simulink model "Simple_Model_Packaging_2"  (R2022b)
settings: Solver=VariableStepAuto  StartTime=0.0  StopTime=0.3  RelTol=1e-3
InitFcn:
  | Parameter_Initialize_2
undefined symbols (not defined in the file or in its folder): doppler, gcbh, magnitude, model, rcfiltgaincompat, rsgenpoly
libraries: commdigbbndpm3 x6, commfilt2 x6, simulink x5, commdigbbndam3 x4, commchan3 x3, commrandsrc3 x3, commblkcod2 x2, commblkintrlv2 x2, commofdm x2, commmimo x2, commseqgen3 x2, commsink2 x1
(part 1 of 2)
settings Model: Creator=89778  LastModifiedBy=79327

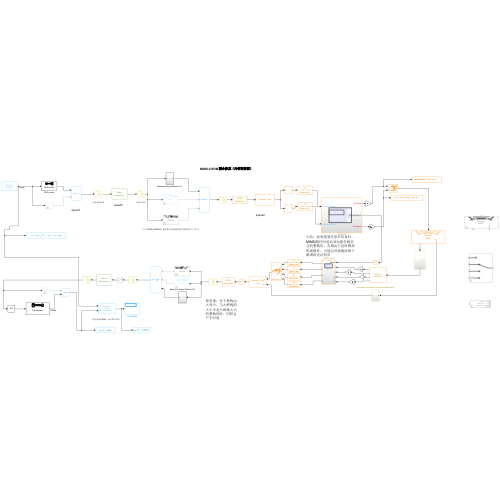
[thumbnail: Simulink's stored preview of the top-level diagram]
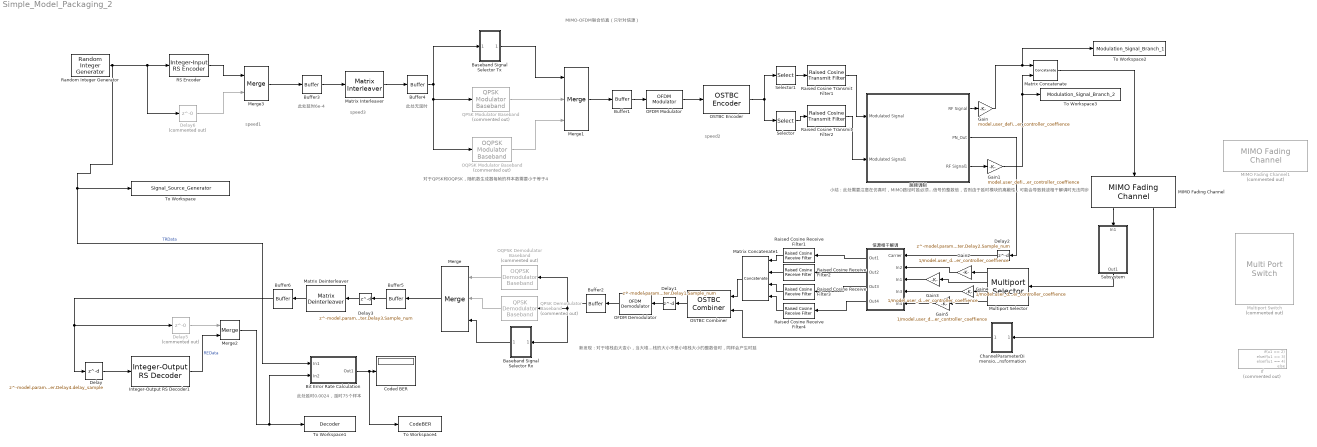
== system Simple_Model_Packaging_2 ==
  note: speed2
  note: 对于QPSK和OQPSK，随机数生成器每帧的样本数需要小于等于4
  note: MIMO-OFDM联合仿真（只针对信源）
  note: 此处延时6e-4
  note: 此处无延时
  note: 此处延时0.0024，延时75个样本
  note: 新发现：对于堆栈由大变小，当大堆栈的大小不是小堆栈大小的整数倍时，同样会产生时延
  note: 小结：此处需要注意在仿真时，MIMO路径时延必须为蓝色线信号的整数倍，否则由于延时模块的离散性，可能会导致载波相干解调时无法同步
  note: speed1
  note: speed3
  Baseband Signal Selector Rx : Subsystem
  Baseband Signal Selector Tx : Subsystem
  Bit Error Rate Calculation : Subsystem
      mask Display:
      | disp('Bit Error\nRate\nCalculation')
      | port_label('input', 1, 'Tx')
      | port_label('input', 2, 'Rx')
  Buffer1 : Buffer  N=model.parameter.Buffer1.Output_size  OutputFrames=off
  Buffer2 : Buffer  N=model.parameter.Buffer2.Output_buffer_size  OutputFrames=off
  Buffer3 : Buffer  N=model.parameter.Buffer3.Output_size  OutputFrames=off
  Buffer4 : Buffer  N=model.parameter.Buffer4.Output_size  OutputFrames=off
  Buffer5 : Buffer  N=model.parameter.Buffer5.Output_buffer_size  OutputFrames=off
  Buffer6 : Buffer  N=model.parameter.Buffer6.Output_buffer_size  OutputFrames=off
  ChannelParameterDimensionTransformation : Subsystem
  Coded BER : Display
  Delay : Delay  DelayLength=model.parameter.Delay4.delay_sample  InitialCondition=0  InputProcessing=Columns as channels (frame based)
  Delay1 : Delay  DelayLength=model.parameter.Delay1.Sample_num  InitialCondition=0  InputProcessing=Columns as channels (frame based)
  Delay2 : Delay  DelayLength=model.parameter.Delay2.Sample_num  InitialCondition=0  InputProcessing=Columns as channels (frame based)
  Delay3 : Delay  DelayLength=model.parameter.Delay3.Sample_num  InitialCondition=0  InputProcessing=Columns as channels (frame based)
  Delay5 : Delay  Commented=on  DelayLength=0  InitialCondition=0  InputProcessing=Columns as channels (frame based)
  Delay6 : Delay  Commented=on  DelayLength=0  InitialCondition=0
  Gain : Gain  Gain=model.user_defined.TR.Sig_power_controller_coeffience
  Gain1 : Gain  Gain=model.user_defined.TR.Sig_power_controller_coeffience
  Gain{2..5} (4 alike) : Gain  Gain=1/model.user_defined.TR.Sig_power_controller_coeffience
  If : If  Commented=on  IfExpression=u1 == 2  ElseIfExpressions=u1 == 3, u1 == 4
  Integer-Output RS Decoder1 : commblkcod2/Integer-Output RS Decoder  n=model.parameter.Integer_Output_RS_Decoder1.Codeword_Length  k=model.parameter.Integer_Output_RS_Decoder1.Message_Length  specShortening=off  shortenedK=3  specGenPoly=off  genPoly=rsgenpoly(7, 3, [], [], 'double')  specPrimPoly=off  prPoly='X^3 + X + 1'  specPuncture=off  punctVec=[ones(2,1); zeros(2,1)]  specErasurePort=off  showNumErr=off
  MIMO Fading Channel : commchan3/MIMO Fading Channel  InheritSampleRate=on  SampleRate=1  PathDelays=model.parameter.MIMO_Fading_Channel.Discrete_path_delays  AveragePathGains=model.parameter.MIMO_Fading_Channel.Average_path_gains  NormalizePathGains=on  FadingDistribution=Rayleigh  KFactor=3  DirectPathDopplerShift=0  DirectPathInitialPhase=0  MaximumDopplerShift=model.parameter.MIMO_Fading_Channel.Maximum_Doppler_shift  DopplerSpectrum=doppler('Jakes')  SpatialCorrelationSpecification=None  SpatialCorrelationMatrix=[1 0 0 0; 0 1 0 0; 0 0 1 0; 0 0 0 1]  NumTransmitAntennas=model.parameter.MIMO_Fading_Channel.TA_num  NumReceiveAntennas=model.parameter.MIMO_Fading_Channel.RA_num  TransmitCorrelationMatrix=[1 0; 0 1]  ReceiveCorrelationMatrix=[1 0; 0 1]  AntennaSelection=Off  NormalizeChannelOutputs=on  PathGainsOutputPort=on  SimulateUsing=Interpreted execution  FadingTechnique=Filtered Gaussian noise  NumSinusoids=48  InitialTimeSource=Property  InitialTime=0  RandomStream=mt19937ar with seed  Seed=73  Visualization=Off  AntennaPairsToDisplay=[ 1, 1 ]  PathsForDopplerDisplay=1  SamplesToDisplay=25%
  MIMO Fading Channel1 : commchan3/MIMO Fading Channel  Commented=on  InheritSampleRate=on  SampleRate=1  PathDelays=[0.000265 0.000265*5]  AveragePathGains=[5 5]  NormalizePathGains=on  FadingDistribution=Rayleigh  KFactor=3  DirectPathDopplerShift=0  DirectPathInitialPhase=0  MaximumDopplerShift=50  DopplerSpectrum=doppler('Jakes')  SpatialCorrelationSpecification=None  SpatialCorrelationMatrix=[1 0 0 0; 0 1 0 0; 0 0 1 0; 0 0 0 1]  NumTransmitAntennas=2  NumReceiveAntennas=2  TransmitCorrelationMatrix=[1 0; 0 1]  ReceiveCorrelationMatrix=[1 0; 0 1]  AntennaSelection=Off  NormalizeChannelOutputs=on  PathGainsOutputPort=on  SimulateUsing=Interpreted execution  FadingTechnique=Filtered Gaussian noise  NumSinusoids=48  InitialTimeSource=Property  InitialTime=0  RandomStream=mt19937ar with seed  Seed=73  Visualization=Off  AntennaPairsToDisplay=[ 1, 1 ]  PathsForDopplerDisplay=1  SamplesToDisplay=25%
  Matrix Concatenate : Concatenate  NumInputs=model.parameter.Matrix_Concatenate.Input_num  Mode=Multidimensional array  ConcatenateDimension=model.parameter.Matrix_Concatenate.Cascade_Dimension
  Matrix Concatenate1 : Concatenate  NumInputs=model.parameter.Matrix_Concatenate1.Input_num  Mode=Multidimensional array  ConcatenateDimension=model.parameter.Matrix_Concatenate1.Cascade_Dimension
  Matrix Deinterleaver : commblkintrlv2/Matrix Deinterleaver  StatePerturbationForJacobian=1.0e-05  Nrows=model.parameter.Matrix_Deinterleaver.row_num  Ncols=model.parameter.Matrix_Deinterleaver.col_num
  Matrix Interleaver : commblkintrlv2/Matrix Interleaver  StatePerturbationForJacobian=1.0e-05  Nrows=model.parameter.Matrix_Interleaver.row_nums  Ncols=model.parameter.Matrix_Interleaver.col_nums
  Merge : Merge  Inputs=3
  Merge1 : Merge  Inputs=3
  Merge2 : Merge
  Merge3 : Merge
  Multiport Selector : dspindex/Multiport Selector  rowsOrCols=Columns  idxCellArray=model.parameter.Multiport_Selector.Indices_to_output  idxErrMode=Clip Index
  Multiport Switch : MultiPortSwitch  Commented=on  SaturateOnIntegerOverflow=off  InputSameDT=off
  OFDM Demodulator : commofdm/OFDM Demodulator  FFTLength=model.parameter.OFDM_Demodulator.FFT_length  NumGuardBandCarriers=model.parameter.OFDM_Demodulator.Number_of_guard_bands  RemoveDCCarrier=off  PilotOutputPort=off  PilotCarrierIndices=[12; 26; 40; 54]  CyclicPrefixLength=model.parameter.OFDM_Demodulator.Cyclic_prefix_length  NumSymbols=model.parameter.OFDM_Demodulator.Number_of_OFDM_symbols  NumReceiveAntennas=model.parameter.OFDM_Demodulator.Number_of_receive_antennas  SimulateUsing=Interpreted execution
  OFDM Modulator : commofdm/OFDM Modulator  StatePerturbationForJacobian=1.0e-05  FFTLength=model.parameter.OFDM_Modulator.FFT_length  NumGuardBandCarriers=model.parameter.OFDM_Modulator.guard_bands_num  InsertDCNull=off  PilotInputPort=off  PilotCarrierIndices=[12; 26; 40; 54]  CyclicPrefixLength=model.parameter.OFDM_Modulator.Cyclic_prefix_length  Windowing=off  WindowLength=1  NumSymbols=model.parameter.OFDM_Modulator.OFDM_symbols_num  NumTransmitAntennas=model.parameter.OFDM_Modulator.transmit_antennas_num  SimulateUsing=Interpreted execution
  OQPSK Demodulator Baseband : commdigbbndpm3/OQPSK Demodulator Baseband  Commented=on  OutType=Integer  Ph=0  Mapping=Gray  pulseShape=Half sine  num=[0.7071, 0.7071]  rolloff=0.2  filterSpan=10  sps=2  RateOptions=Enforce single-rate processing  outDtype2=double
  OQPSK Modulator Baseband : commdigbbndpm3/OQPSK Modulator Baseband  Commented=on  InType=Integer  Ph=0  Mapping=Gray  pulseShape=Half sine  num=[0.7071, 0.7071]  rolloff=0.2  filterSpan=10  sps=2  RateOptions=Enforce single-rate processing  outDtype=double
  OSTBC Combiner : commmimo/OSTBC Combiner  numTx=2  rate=3/4  numRx=4  roundingMode=Floor  overflowMode=Wrap  OvFlMode=off  OvFlModeLastStrValue=off  crossProductWordLen=32  crossProductFracLen=16  crossSumWordLen=32  crossSumFracLen=16  egyProductWordLen=32  egyProductFracLen=16  egySumWordLen=32  egySumFracLen=16  divisionWordLen=32  divisionFracLen=16  divisionDataTypeStr=Inherit: Same as accumulator  divisionLastDataTypeStr=Inherit: Same as accumulator
  OSTBC Encoder : commmimo/OSTBC Encoder  numTx=2  rate=3/4  overflowMode=Wrap  OvFlMode=off  OvFlModeLastStrValue=off
  QPSK Demodulator Baseband : commdigbbndpm3/QPSK Demodulator Baseband  Commented=on  OutType=Integer  DecType=Hard decision  VarSource=Dialog  Variance=1  Dec=Gray  Ph=pi/4  outDtype1=Inherit via internal rule  outDtype2=Inherit via internal rule  derotateFactorWordLen=16  derotateFactorDataTypeStr=Inherit: Same word length as input  derotateFactorLastDataTypeStr=Inherit: Same word length as input
  QPSK Modulator Baseband : commdigbbndpm3/QPSK Modulator Baseband  Commented=on  InType=Integer  Enc=Gray  Ph=pi/4  outDtype=double  outWordLen=16  outUDDataType=sfix(16)  outFracLenMode=Best precision  outFracLen=15  outDataTypeStr=double  outLastDataTypeStr=double
  RS Encoder : commblkcod2/Integer-Input RS Encoder  n=model.parameter.RS_Encoder.Codeword_Length  k=model.parameter.RS_Encoder.Message_Length  specShortening=off  shortenedK=3  specGenPoly=off  genPoly=rsgenpoly(7,3)  specPrimPoly=off  prPoly=[1 0 1 1]  specPuncture=off  punctVec=[ones(2,1); zeros(2,1)]
  Raised Cosine Receive Filter1 : commfilt2/Raised Cosine Receive Filter  filtType=Square root  R=model.parameter.Raised_Cosine_Receive_Filter1.Rolloff_factor  filtSpan=model.parameter.Raised_Cosine_Receive_Filter1.Filter_span_in_symbols  N=model.parameter.Raised_Cosine_Receive_Filter1.Input_samples_per_symbol  downFactor=model.parameter.Raised_Cosine_Receive_Filter1.Decimation_factor  downOffset=0  filterGain=rcfiltgaincompat(gcbh)  InputProcessing=Columns as channels (frame based)  RateOptions=Enforce single-rate processing  framing=Mute  checkCoeff=off  variableName=rcRxFilt1  currentFiltSpan=10  D=5  inputOffset=0  sampMode=Mute  saveAsFlag=0  rateMode=Downsampling  checkGain=Normalized  launchFVT=on  roundingMode=Floor  overflowMode=off  coeffDataTypeStr=Inherit: Same word length as input  coeffMin=[]  coeffMax=[]  coeffLastDataTypeStr=Inherit: Same word length as input  accumDataTypeStr=Inherit: Same as product output  accumLastDataTypeStr=Inherit: Same as product output  outputDataTypeStr=Inherit: Same as accumulator  outputMin=[]  outputMax=[]  outputLastDataTypeStr=Inherit: Same as accumulator
  Raised Cosine Receive Filter2 : commfilt2/Raised Cosine Receive Filter  filtType=Square root  R=model.parameter.Raised_Cosine_Receive_Filter2.Rolloff_factor  filtSpan=model.parameter.Raised_Cosine_Receive_Filter2.Filter_span_in_symbols  N=model.parameter.Raised_Cosine_Receive_Filter2.Input_samples_per_symbol  downFactor=model.parameter.Raised_Cosine_Receive_Filter2.Decimation_factor  downOffset=0  filterGain=rcfiltgaincompat(gcbh)  InputProcessing=Columns as channels (frame based)  RateOptions=Enforce single-rate processing  framing=Mute  checkCoeff=off  variableName=rcRxFilt2  currentFiltSpan=10  D=5  inputOffset=0  sampMode=Mute  saveAsFlag=0  rateMode=Downsampling  checkGain=Normalized  launchFVT=on  roundingMode=Floor  overflowMode=off  coeffDataTypeStr=Inherit: Same word length as input  coeffMin=[]  coeffMax=[]  coeffLastDataTypeStr=Inherit: Same word length as input  accumDataTypeStr=Inherit: Same as product output  accumLastDataTypeStr=Inherit: Same as product output  outputDataTypeStr=Inherit: Same as accumulator  outputMin=[]  outputMax=[]  outputLastDataTypeStr=Inherit: Same as accumulator
  Raised Cosine Receive Filter3 : commfilt2/Raised Cosine Receive Filter  filtType=Square root  R=model.parameter.Raised_Cosine_Receive_Filter2.Rolloff_factor  filtSpan=model.parameter.Raised_Cosine_Receive_Filter2.Filter_span_in_symbols  N=model.parameter.Raised_Cosine_Receive_Filter2.Input_samples_per_symbol  downFactor=model.parameter.Raised_Cosine_Receive_Filter2.Decimation_factor  downOffset=0  filterGain=rcfiltgaincompat(gcbh)  InputProcessing=Columns as channels (frame based)  RateOptions=Enforce single-rate processing  framing=Mute  checkCoeff=off  variableName=rcRxFilt3  currentFiltSpan=10  D=5  inputOffset=0  sampMode=Mute  saveAsFlag=0  rateMode=Downsampling  checkGain=Normalized  launchFVT=on  roundingMode=Floor  overflowMode=off  coeffDataTypeStr=Inherit: Same word length as input  coeffMin=[]  coeffMax=[]  coeffLastDataTypeStr=Inherit: Same word length as input  accumDataTypeStr=Inherit: Same as product output  accumLastDataTypeStr=Inherit: Same as product output  outputDataTypeStr=Inherit: Same as accumulator  outputMin=[]  outputMax=[]  outputLastDataTypeStr=Inherit: Same as accumulator
  Raised Cosine Receive Filter4 : commfilt2/Raised Cosine Receive Filter  filtType=Square root  R=model.parameter.Raised_Cosine_Receive_Filter2.Rolloff_factor  filtSpan=model.parameter.Raised_Cosine_Receive_Filter2.Filter_span_in_symbols  N=model.parameter.Raised_Cosine_Receive_Filter2.Input_samples_per_symbol  downFactor=model.parameter.Raised_Cosine_Receive_Filter2.Decimation_factor  downOffset=0  filterGain=rcfiltgaincompat(gcbh)  InputProcessing=Columns as channels (frame based)  RateOptions=Enforce single-rate processing  framing=Mute  checkCoeff=off  variableName=rcRxFilt4  currentFiltSpan=10  D=5  inputOffset=0  sampMode=Mute  saveAsFlag=0  rateMode=Downsampling  checkGain=Normalized  launchFVT=on  roundingMode=Floor  overflowMode=off  coeffDataTypeStr=Inherit: Same word length as input  coeffMin=[]  coeffMax=[]  coeffLastDataTypeStr=Inherit: Same word length as input  accumDataTypeStr=Inherit: Same as product output  accumLastDataTypeStr=Inherit: Same as product output  outputDataTypeStr=Inherit: Same as accumulator  outputMin=[]  outputMax=[]  outputLastDataTypeStr=Inherit: Same as accumulator
  Raised Cosine Transmit Filter1 : commfilt2/Raised Cosine Transmit Filter  filtType=Square root  R=model.parameter.Raised_Cosine_Transmit_Filter1.Rolloff_factor  filtSpan=model.parameter.Raised_Cosine_Transmit_Filter1.Filter_span_in_symbols  N=model.parameter.Raised_Cosine_Transmit_Filter1.Output_samples_per_symbol  filterGain=rcfiltgaincompat(gcbh)  InputProcessing=Columns as channels (frame based)  RateOptions=Enforce single-rate processing  framing=Mute  checkCoeff=off  variableName=rcTxFilt1  checkGain=Normalized  sampMode=Mute  saveAsFlag=0  currentFiltSpan=10  D=(10)/2  launchFVT=on  roundingMode=Floor  overflowMode=off  coeffDataTypeStr=Inherit: Same word length as input  coeffMin=[]  coeffMax=[]  coeffLastDataTypeStr=Inherit: Same word length as input  outputDataTypeStr=Inherit: Same as accumulator  outputMin=[]  outputMax=[]  outputLastDataTypeStr=Inherit: Same as accumulator
  Raised Cosine Transmit Filter2 : commfilt2/Raised Cosine Transmit Filter  filtType=Square root  R=model.parameter.Raised_Cosine_Transmit_Filter2.Rolloff_factor  filtSpan=model.parameter.Raised_Cosine_Transmit_Filter2.Filter_span_in_symbols  N=model.parameter.Raised_Cosine_Transmit_Filter2.Output_samples_per_symbol  filterGain=rcfiltgaincompat(gcbh)  InputProcessing=Columns as channels (frame based)  RateOptions=Enforce single-rate processing  framing=Mute  checkCoeff=off  variableName=rcTxFilt2  checkGain=Normalized  sampMode=Mute  saveAsFlag=0  currentFiltSpan=10  D=(10)/2  launchFVT=on  roundingMode=Floor  overflowMode=off  coeffDataTypeStr=Inherit: Same word length as input  coeffMin=[]  coeffMax=[]  coeffLastDataTypeStr=Inherit: Same word length as input  outputDataTypeStr=Inherit: Same as accumulator  outputMin=[]  outputMax=[]  outputLastDataTypeStr=Inherit: Same as accumulator
  Random Integer Generator : commrandsrc3/Random Integer Generator  SetSize=model.parameter.Random_Integer_Generator.SetSize  SeedSource=Auto  Seed=4  SampleTime=model.parameter.Random_Integer_Generator.Random_Sample_Time  SamplesPerFrame=model.parameter.Random_Integer_Generator.Samples_per_frame  OutputDataType=double  SimulateUsing=Interpreted execution
  Selector : Selector  NumberOfDimensions=2  InputPortWidth=3  IndexOptions=Index vector (dialog),Index vector (dialog)  Indices=[1:272],2  OutputSizes=1,1
  Selector1 : Selector  NumberOfDimensions=2  InputPortWidth=3  IndexOptions=Index vector (dialog),Index vector (dialog)  Indices=[1:272],1  OutputSizes=1,1
  Subsystem : Subsystem
  To Workspace : ToWorkspace  VariableName=Signal_Source_Generator  SaveFormat=Timeseries  SampleTime=-1
  To Workspace1 : ToWorkspace  VariableName=Decoder  SaveFormat=Timeseries  SampleTime=-1
  To Workspace2 : ToWorkspace  VariableName=Modulation_Signal_Branch_1  SaveFormat=Timeseries  SampleTime=-1
  To Workspace3 : ToWorkspace  VariableName=Modulation_Signal_Branch_2  SaveFormat=Timeseries  SampleTime=-1
  To Workspace4 : ToWorkspace  VariableName=CodeBER  SaveFormat=Timeseries  SampleTime=-1
  信源相干解调 : Subsystem
  跳频调制 : Subsystem
  wires:
  Selector/1 -> Raised Cosine Transmit Filter2/1
  Selector1/1 -> Raised Cosine Transmit Filter1/1
  Matrix Interleaver/1 -> Buffer4/1
  Buffer3/1 -> Matrix Interleaver/1
  Buffer1/1 -> OFDM Modulator/1
  OFDM Modulator/1 -> OSTBC Encoder/1
  OSTBC Encoder/1 -> Selector1/1, Selector/1
  Raised Cosine Transmit Filter1/1 -> 跳频调制/1(Modulated Signal)
  Raised Cosine Transmit Filter2/1 -> 跳频调制/2(Modulated Signal1)
  跳频调制/1(RF Signal) -> Gain/1
  跳频调制/3(RF Signal1) -> Gain1/1
  Delay2/1 -> 信源相干解调/1(Carrier)
  信源相干解调/2(Out2) -> Raised Cosine Receive Filter2/1
  MIMO Fading Channel/2 -> ChannelParameterDimensionTransformation/1(In1)
  OFDM Demodulator/1 -> Buffer2/1
  Bit Error Rate Calculation/1(Out1) -> To Workspace4/1, Coded BER/1
  Raised Cosine Receive Filter1/1 -> Matrix Concatenate1/1
  Multiport Selector/1 -> Gain2/1
  Multiport Selector/2 -> Gain3/1
  Matrix Deinterleaver/1 -> Buffer6/1
  信源相干解调/1(Out1) -> Raised Cosine Receive Filter1/1
  OSTBC Combiner/1 -> Delay1/1
  Delay3/1 -> Matrix Deinterleaver/1
  Matrix Concatenate1/1 -> OSTBC Combiner/1
  ChannelParameterDimensionTransformation/1(Out1) -> OSTBC Combiner/2
  Raised Cosine Receive Filter2/1 -> Matrix Concatenate1/2
  Delay1/1 -> OFDM Demodulator/1
  跳频调制/2(PN_Out) -> Delay2/1
  MIMO Fading Channel/1 -> Subsystem/1(In1)
  Subsystem/1(Out1) -> Multiport Selector/1
  Multiport Selector/3 -> Gain4/1
  Multiport Selector/4 -> Gain5/1
  信源相干解调/3(Out3) -> Raised Cosine Receive Filter3/1
  信源相干解调/4(Out4) -> Raised Cosine Receive Filter4/1
  Raised Cosine Receive Filter3/1 -> Matrix Concatenate1/3
  Raised Cosine Receive Filter4/1 -> Matrix Concatenate1/4
  QPSK Modulator Baseband/1 -> Merge1/2
  Random Integer Generator/1 -> RS Encoder/1, Delay6/1, To Workspace/1, Bit Error Rate Calculation/1(In1)  "TRData"
  Baseband Signal Selector Tx/1(Out1) -> Merge1/1
  OQPSK Modulator Baseband/1 -> Merge1/3
  Delay5/1 -> Merge2/1
  Delay/1 -> Integer-Output RS Decoder1/1
  Integer-Output RS Decoder1/1 -> Merge2/2  "REData"
  Merge2/1 -> To Workspace1/1, Bit Error Rate Calculation/2(In2)
  Buffer4/1 -> Baseband Signal Selector Tx/1(In1), QPSK Modulator Baseband/1, OQPSK Modulator Baseband/1
  Merge1/1 -> Buffer1/1
  RS Encoder/1 -> Merge3/1
  Delay6/1 -> Merge3/2
  Merge3/1 -> Buffer3/1
  Buffer6/1 -> Delay/1, Delay5/1
  Buffer5/1 -> Delay3/1
  Buffer2/1 -> OQPSK Demodulator Baseband/1, Baseband Signal Selector Rx/1(In1), QPSK Demodulator Baseband/1
  OQPSK Demodulator Baseband/1 -> Merge/1
  QPSK Demodulator Baseband/1 -> Merge/2
  Baseband Signal Selector Rx/1(Out1) -> Merge/3
  Merge/1 -> Buffer5/1
  Gain/1 -> To Workspace2/1, Matrix Concatenate/1
  Gain1/1 -> Matrix Concatenate/2, To Workspace3/1
  Gain2/1 -> 信源相干解调/2(In2)
  Gain3/1 -> 信源相干解调/3(In1)
  Gain4/1 -> 信源相干解调/4(In3)
  Gain5/1 -> 信源相干解调/5(In4)
  Matrix Concatenate/1 -> MIMO Fading Channel/1

== system Simple_Model_Packaging_2/Baseband Signal Selector Rx ==
  In1 : Inport
  Constant : Constant  Value=model.user_defined.TR.Baseband_Modulation_type
  If : If  IfExpression=u1 == 1  ElseIfExpressions=u1 == 2
  If Action Subsystem1 : Subsystem  TreatAsAtomicUnit=on
  If Action Subsystem4 : Subsystem  TreatAsAtomicUnit=on
  If Action Subsystem5 : Subsystem  TreatAsAtomicUnit=on
  Merge : Merge  Inputs=3
  Out1 : Outport
  wires:
  In1/1 -> If Action Subsystem4/1(In1), If Action Subsystem1/1(In1), If Action Subsystem5/1(In1)
  If Action Subsystem5/1(Out1) -> Merge/3
  If Action Subsystem1/1(Out1) -> Merge/2
  If Action Subsystem4/1(Out1) -> Merge/1
  Constant/1 -> If/1
  Merge/1 -> Out1/1
  If/3 -> If Action Subsystem5/Action
  If/1 -> If Action Subsystem4/Action
  If/2 -> If Action Subsystem1/Action

== system Simple_Model_Packaging_2/Baseband Signal Selector Tx ==
  In1 : Inport
  Constant : Constant  Value=model.user_defined.TR.Baseband_Modulation_type
  If : If  IfExpression=u1 == 1  ElseIfExpressions=u1 == 2
  If Action Subsystem1 : Subsystem  TreatAsAtomicUnit=on
  If Action Subsystem4 : Subsystem  TreatAsAtomicUnit=on
  If Action Subsystem5 : Subsystem  TreatAsAtomicUnit=on
  Merge : Merge  Inputs=3
  Out1 : Outport
  wires:
  If Action Subsystem5/1(Out1) -> Merge/3
  Constant/1 -> If/1
  Merge/1 -> Out1/1
  If/3 -> If Action Subsystem5/Action
  If/1 -> If Action Subsystem4/Action
  If/2 -> If Action Subsystem1/Action
  If Action Subsystem1/1(Out1) -> Merge/2
  If Action Subsystem4/1(Out1) -> Merge/1
  In1/1 -> If Action Subsystem4/1(In1), If Action Subsystem1/1(In1), If Action Subsystem5/1(In1)

== system Simple_Model_Packaging_2/Bit Error Rate Calculation ==
  In1 : Inport
  In2 : Inport  Port=2
  Error Rate Calculation : commsink2/Error Rate Calculation  N=model.parameter.Error_Rate_Calculation.Receive_delay  st_delay=0  cp_mode=Entire frame  subframe=[]  PMode=Port  WsName=ErrorVec  RsMode2=off  stop=on  numErr=1e8  maxBits=1e10
  Integer to Bit Converter : simulink/Logic and Bit Operations/Integer to Bit Converter  nbits=model.parameter.Integer_to_Bit_Converter.M  signedInputValues=Unsigned  bitOrder=MSB first  outDtype=Inherit via internal rule
      settings: LibrarySourceBlock=|
      | commutil2/Integer to Bit
      | Converter
  Integer to Bit Converter1 : simulink/Logic and Bit Operations/Integer to Bit Converter  nbits=model.parameter.Integer_to_Bit_Converter1.M  signedInputValues=Unsigned  bitOrder=MSB first  outDtype=Inherit via internal rule
      settings: LibrarySourceBlock=|
      | commutil2/Integer to Bit
      | Converter
  Out1 : Outport  VectorParamsAs1DForOutWhenUnconnected=off
  wires:
  Integer to Bit Converter/1 -> Error Rate Calculation/1
  Integer to Bit Converter1/1 -> Error Rate Calculation/2
  In1/1 -> Integer to Bit Converter/1
  Error Rate Calculation/1 -> Out1/1
  In2/1 -> Integer to Bit Converter1/1

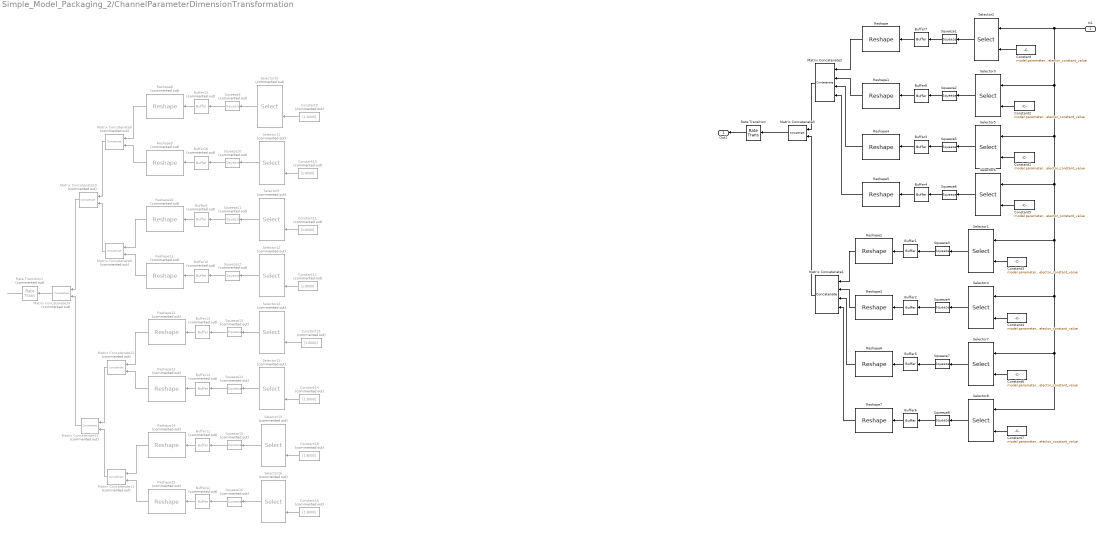
== system Simple_Model_Packaging_2/ChannelParameterDimensionTransformation ==
  In1 : Inport
  Buffer{1..8} (8 alike) : Buffer  N=model.parameter.CSI.buffers_length  OutputFrames=off
  Buffer{9..16} (8 alike) : Buffer  Commented=on  N=80  OutputFrames=off
  Constant{,1..7} (8 alike) : Constant  Value=model.parameter.CSI.selector_constant_value
  Constant{9..16} (8 alike) : Constant  Commented=on  Value=[1:8000]
  Matrix Concatenate1 : Concatenate  NumInputs=4  Mode=Multidimensional array  ConcatenateDimension=3
  Matrix Concatenate10 : Concatenate  Commented=on  Mode=Multidimensional array  ConcatenateDimension=3
  Matrix Concatenate{8..9,11..12} (4 alike) : Concatenate  Commented=on  Mode=Multidimensional array  ConcatenateDimension=4
  Matrix Concatenate13 : Concatenate  Commented=on  Mode=Multidimensional array  ConcatenateDimension=3
  Matrix Concatenate14 : Concatenate  Commented=on  Mode=Multidimensional array  ConcatenateDimension=2
  Matrix Concatenate2 : Concatenate  NumInputs=4  Mode=Multidimensional array  ConcatenateDimension=3
  Matrix Concatenate3 : Concatenate  Mode=Multidimensional array  ConcatenateDimension=2
  Rate Transition : RateTransition  OutPortSampleTime=model.Intermediate_variable.system_frame_speed_2
  Rate Transition1 : RateTransition  Commented=on  OutPortSampleTime=2.65e-4
  Reshape{,1..7} (8 alike) : Reshape  OutputDimensionality=Customize  OutputDimensions=model.parameter.CSI.reshape_dimension
  Reshape{8..15} (8 alike) : Reshape  Commented=on  OutputDimensionality=Customize  OutputDimensions=[80,1,1,1]
  Selector1 : Selector  NumberOfDimensions=4  InputPortWidth=3  IndexOptions=Index vector (port),Index vector (dialog),Index vector (dialog),Index vector (dialog)  Indices=[1 3],1,2,1  OutputSizes=1,1,1,1
  Selector10 : Selector  Commented=on  NumberOfDimensions=4  InputPortWidth=3  IndexOptions=Index vector (port),Index vector (dialog),Index vector (dialog),Index vector (dialog)  Indices=[1 3],1,1,1  OutputSizes=1,1,1,1
  Selector11 : Selector  Commented=on  NumberOfDimensions=4  InputPortWidth=3  IndexOptions=Index vector (port),Index vector (dialog),Index vector (dialog),Index vector (dialog)  Indices=[1 3],1,1,2  OutputSizes=1,1,1,1
  Selector12 : Selector  Commented=on  NumberOfDimensions=4  InputPortWidth=3  IndexOptions=Index vector (port),Index vector (dialog),Index vector (dialog),Index vector (dialog)  Indices=[1 3],1,2,2  OutputSizes=1,1,1,1
  Selector13 : Selector  Commented=on  NumberOfDimensions=4  InputPortWidth=3  IndexOptions=Index vector (port),Index vector (dialog),Index vector (dialog),Index vector (dialog)  Indices=[1 3],2,2,1  OutputSizes=1,1,1,1
  Selector14 : Selector  Commented=on  NumberOfDimensions=4  InputPortWidth=3  IndexOptions=Index vector (port),Index vector (dialog),Index vector (dialog),Index vector (dialog)  Indices=[1 3],2,1,1  OutputSizes=1,1,1,1
  Selector15 : Selector  Commented=on  NumberOfDimensions=4  InputPortWidth=3  IndexOptions=Index vector (port),Index vector (dialog),Index vector (dialog),Index vector (dialog)  Indices=[1 3],2,1,2  OutputSizes=1,1,1,1
  Selector16 : Selector  Commented=on  NumberOfDimensions=4  InputPortWidth=3  IndexOptions=Index vector (port),Index vector (dialog),Index vector (dialog),Index vector (dialog)  Indices=[1 3],2,2,2  OutputSizes=1,1,1,1
  Selector2 : Selector  NumberOfDimensions=4  InputPortWidth=3  IndexOptions=Index vector (port),Index vector (dialog),Index vector (dialog),Index vector (dialog)  Indices=[1 3],1,1,1  OutputSizes=1,1,1,1
  Selector3 : Selector  NumberOfDimensions=4  InputPortWidth=3  IndexOptions=Index vector (port),Index vector (dialog),Index vector (dialog),Index vector (dialog)  Indices=[1 3],1,1,2  OutputSizes=1,1,1,1
  Selector4 : Selector  NumberOfDimensions=4  InputPortWidth=3  IndexOptions=Index vector (port),Index vector (dialog),Index vector (dialog),Index vector (dialog)  Indices=[1 3],1,2,2  OutputSizes=1,1,1,1
  Selector5 : Selector  NumberOfDimensions=4  InputPortWidth=3  IndexOptions=Index vector (port),Index vector (dialog),Index vector (dialog),Index vector (dialog)  Indices=[1 3],1,1,3  OutputSizes=1,1,1,1
  Selector6 : Selector  NumberOfDimensions=4  InputPortWidth=3  IndexOptions=Index vector (port),Index vector (dialog),Index vector (dialog),Index vector (dialog)  Indices=[1 3],1,1,4  OutputSizes=1,1,1,1
  Selector7 : Selector  NumberOfDimensions=4  InputPortWidth=3  IndexOptions=Index vector (port),Index vector (dialog),Index vector (dialog),Index vector (dialog)  Indices=[1 3],1,2,3  OutputSizes=1,1,1,1
  Selector8 : Selector  NumberOfDimensions=4  InputPortWidth=3  IndexOptions=Index vector (port),Index vector (dialog),Index vector (dialog),Index vector (dialog)  Indices=[1 3],1,2,4  OutputSizes=1,1,1,1
  Selector9 : Selector  Commented=on  NumberOfDimensions=4  InputPortWidth=3  IndexOptions=Index vector (port),Index vector (dialog),Index vector (dialog),Index vector (dialog)  Indices=[1 3],1,2,1  OutputSizes=1,1,1,1
  Squeeze{1..8} (8 alike) : Squeeze
  Squeeze{9..16} (8 alike) : Squeeze  Commented=on
  Out1 : Outport
  wires:
  Buffer8/1 -> Reshape1/1
  Buffer7/1 -> Reshape/1
  Squeeze2/1 -> Buffer8/1
  Constant2/1 -> Selector3/2
  Selector3/1 -> Squeeze2/1
  Constant/1 -> Selector2/2
  Selector2/1 -> Squeeze1/1
  Reshape/1 -> Matrix Concatenate2/1
  Squeeze1/1 -> Buffer7/1
  Reshape1/1 -> Matrix Concatenate2/2
  Selector1/1 -> Squeeze3/1
  Constant3/1 -> Selector1/2
  Squeeze3/1 -> Buffer1/1
  Selector4/1 -> Squeeze4/1
  Constant4/1 -> Selector4/2
  Squeeze4/1 -> Buffer2/1
  Buffer1/1 -> Reshape2/1
  Buffer2/1 -> Reshape3/1
  Reshape2/1 -> Matrix Concatenate1/1
  Reshape3/1 -> Matrix Concatenate1/2
  Matrix Concatenate2/1 -> Matrix Concatenate3/1
  Matrix Concatenate1/1 -> Matrix Concatenate3/2
  Rate Transition/1 -> Out1/1
  Matrix Concatenate3/1 -> Rate Transition/1
  Matrix Concatenate8/1 -> Matrix Concatenate10/2
  Squeeze12/1 -> Buffer10/1
  Buffer10/1 -> Reshape11/1
  Constant12/1 -> Selector12/2
  Reshape9/1 -> Matrix Concatenate9/2
  Buffer16/1 -> Reshape9/1
  Selector9/1 -> Squeeze11/1
  Reshape10/1 -> Matrix Concatenate8/1
  Reshape8/1 -> Matrix Concatenate9/1
  Buffer9/1 -> Reshape10/1
  Matrix Concatenate10/1 -> Matrix Concatenate14/1
  Buffer15/1 -> Reshape8/1
  Selector10/1 -> Squeeze9/1
  Constant9/1 -> Selector10/2
  Constant11/1 -> Selector9/2
  Constant10/1 -> Selector11/2
  Constant14/1 -> Selector15/2
  Selector15/1 -> Squeeze14/1
  Squeeze9/1 -> Buffer15/1
  Selector16/1 -> Squeeze16/1
  Selector13/1 -> Squeeze15/1
  Reshape15/1 -> Matrix Concatenate11/2
  Squeeze13/1 -> Buffer13/1
  Selector11/1 -> Squeeze10/1
  Squeeze14/1 -> Buffer14/1
  Buffer14/1 -> Reshape13/1
  Selector14/1 -> Squeeze13/1
  Buffer13/1 -> Reshape12/1
  Buffer11/1 -> Reshape14/1
  Matrix Concatenate13/1 -> Matrix Concatenate14/2
  Buffer12/1 -> Reshape15/1
  Matrix Concatenate11/1 -> Matrix Concatenate13/2
  Constant15/1 -> Selector13/2
  Squeeze16/1 -> Buffer12/1
  Squeeze10/1 -> Buffer16/1
  Reshape13/1 -> Matrix Concatenate12/2
  Matrix Concatenate9/1 -> Matrix Concatenate10/1
  Constant16/1 -> Selector16/2
  Constant13/1 -> Selector14/2
  Selector12/1 -> Squeeze12/1
  Rate Transition1/1 -> ?
  Reshape12/1 -> Matrix Concatenate12/1
  Squeeze15/1 -> Buffer11/1
  ? -> Selector9/1, Selector12/1, Selector16/1, Selector13/1, Selector15/1, Selector14/1, Selector11/1, Selector10/1
  Squeeze11/1 -> Buffer9/1
  Reshape11/1 -> Matrix Concatenate8/2
  Matrix Concatenate14/1 -> Rate Transition1/1
  Matrix Concatenate12/1 -> Matrix Concatenate13/1
  Reshape14/1 -> Matrix Concatenate11/1
  Constant1/1 -> Selector5/2
  Constant5/1 -> Selector6/2
  Squeeze5/1 -> Buffer3/1
  Buffer3/1 -> Reshape4/1
  Squeeze6/1 -> Buffer4/1
  Buffer4/1 -> Reshape5/1
  Selector5/1 -> Squeeze5/1
  Selector6/1 -> Squeeze6/1
  Reshape4/1 -> Matrix Concatenate2/3
  Reshape5/1 -> Matrix Concatenate2/4
  Selector7/1 -> Squeeze7/1
  Buffer5/1 -> Reshape6/1
  Squeeze7/1 -> Buffer5/1
  Constant6/1 -> Selector7/2
  In1/1 -> Selector6/1, Selector1/1, Selector8/1, Selector7/1, Selector4/1, Selector5/1, Selector3/1, Selector2/1
  Selector8/1 -> Squeeze8/1
  Buffer6/1 -> Reshape7/1
  Squeeze8/1 -> Buffer6/1
  Constant7/1 -> Selector8/2
  Reshape6/1 -> Matrix Concatenate1/3
  Reshape7/1 -> Matrix Concatenate1/4

== system Simple_Model_Packaging_2/Subsystem ==
  In1 : Inport
  AWGN Channel : commchan3/AWGN Channel  InputProcessing=Columns as channels (frame based)  seed=67  noiseMode="Signal to noise ratio  (SNR)"  EbNodB=10  EsNodB=10  SNRdB=model.parameter.Awgn.SNR  bitsPerSym=1  Ps=model.parameter.Awgn.input_power  Tsym=1  variance=1
  Add : Sum
  Buffer : Buffer  N=model.parameter.M_FSK_Modulator_Baseband1.Samples_per_symbol  OutputFrames=off
  NosieGen : Subsystem
  Vector Concatenate : Concatenate  NumInputs=4  Mode=Multidimensional array  ConcatenateDimension=2
  Out1 : Outport
  wires:
  In1/1 -> Add/2
  AWGN Channel/1 -> Out1/1
  Add/1 -> AWGN Channel/1  "RESignal"
  Vector Concatenate/1 -> Add/1
  Buffer/1 -> Vector Concatenate/4, Vector Concatenate/3, Vector Concatenate/2, Vector Concatenate/1  "TRSignal"
  NosieGen/1(Jamming_Signal_Output) -> Buffer/1

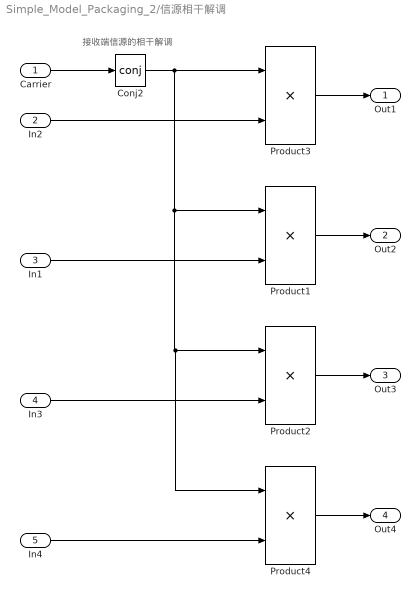
== system Simple_Model_Packaging_2/信源相干解调 ==
  note: 接收端信源的相干解调
  Carrier : Inport
  In2 : Inport  Port=2
  In1 : Inport  Port=3
  In3 : Inport  Port=4
  In4 : Inport  Port=5
  Conj2 : Math  Operator=conj
  Product{1..4} (4 alike) : Product
  Out1 : Outport
  Out2 : Outport  Port=2
  Out3 : Outport  Port=3
  Out4 : Outport  Port=4
  wires:
  Carrier/1 -> Conj2/1
  In2/1 -> Product3/2
  Product3/1 -> Out1/1
  In1/1 -> Product1/2
  Product1/1 -> Out2/1
  Conj2/1 -> Product4/1, Product2/1, Product1/1, Product3/1
  Product2/1 -> Out3/1
  Product4/1 -> Out4/1
  In3/1 -> Product2/2
  In4/1 -> Product4/2

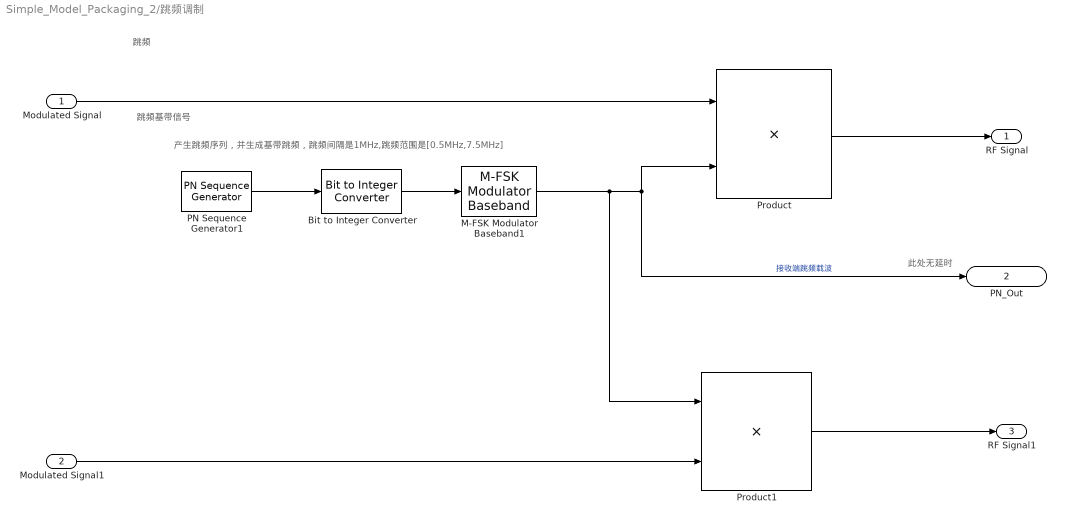
== system Simple_Model_Packaging_2/跳频调制 ==
  note: 跳频
  note: 此处无延时
  note: 跳频基带信号
  note: 产生跳频序列，并生成基带跳频，跳频间隔是1MHz,跳频范围是[0.5MHz,7.5MHz]
  Modulated Signal : Inport
  Modulated Signal1 : Inport  Port=2
  Bit to Integer Converter : simulink/Logic and Bit Operations/Bit to Integer Converter  nbits=model.parameter.Bit_to_Integer_Converter.M  bitOrder=MSB first  signedOutputValues=Unsigned  outDtype=double  outDtypeSigned=Inherit via internal rule
  M-FSK Modulator Baseband1 : commdigbbndfm2/M-FSK Modulator Baseband  M=model.parameter.M_FSK_Modulator_Baseband1.M_ary_number  InType=Integer  Enc=Gray  freqSep=model.parameter.M_FSK_Modulator_Baseband1.Frequency_separation  phaseType=Continuous  numSamp=model.parameter.M_FSK_Modulator_Baseband1.Samples_per_symbol  RateOptions=Enforce single-rate processing  outDataType=double
  PN Sequence Generator1 : commseqgen3/PN Sequence Generator  poly=model.parameter.PN_Sequence_Generator1.Generator_polynomial  ini_sta=model.parameter.PN_Sequence_Generator1.Initial_states  outBitMaskSource=Dialog parameter  shift=0  outVarSiz=off  maxOutSizeMode=Dialog parameter  maxOutSize=[10 1]  Ts=model.parameter.PN_Sequence_Generator1.Sample_time  sampPerFrame=model.parameter.PN_Sequence_Generator1.Samples_per_frame  reset=off  bitPackedOutputs=off  outDataType=double  numPackedBits=5  bitPackDataSigned=off  bitPackedOutDType=double
  Product : Product
  Product1 : Product
  RF Signal : Outport
  PN_Out : Outport  Port=2
  RF Signal1 : Outport  Port=3
  wires:
  M-FSK Modulator Baseband1/1 -> PN_Out/1, Product/2, Product1/1  "接收端跳频载波"
  Product/1 -> RF Signal/1
  Product1/1 -> RF Signal1/1
  Modulated Signal1/1 -> Product1/2
  Modulated Signal/1 -> Product/1
  PN Sequence Generator1/1 -> Bit to Integer Converter/1
  Bit to Integer Converter/1 -> M-FSK Modulator Baseband1/1

== system Simple_Model_Packaging_2/Baseband Signal Selector Rx/If Action Subsystem1 ==
  In1 : Inport
  Action Port : ActionPort  ActionPortLabel=elseif(u1 == 2)
  M-PSK Demodulator Baseband : commdigbbndpm3/M-PSK Demodulator Baseband  M=model.user_defined.Rectangular_QAM_Modulator_Baseband.M_Number  OutType=Integer  DecType=Hard decision  VarSource=Dialog  Variance=1  Dec=Gray  Mapping=[0:7]  Ph=0  outDtype1=Inherit via internal rule  outDtype2=Inherit via internal rule  derotateFactorWordLen=16  derotateFactorDataTypeStr=Inherit: Same word length as input  derotateFactorLastDataTypeStr=Inherit: Same word length as input
  Out1 : Outport
  wires:
  In1/1 -> M-PSK Demodulator Baseband/1
  M-PSK Demodulator Baseband/1 -> Out1/1  "REData"

== system Simple_Model_Packaging_2/Baseband Signal Selector Rx/If Action Subsystem4 ==
  In1 : Inport
  Action Port : ActionPort  ActionPortLabel=if(u1 == 1)
  Rectangular QAM Demodulator Baseband : commdigbbndam3/Rectangular QAM Demodulator Baseband  M=model.user_defined.Rectangular_QAM_Modulator_Baseband.M_Number  OutType=Integer  DecType=Hard decision  VarSource=Dialog  Variance=1  Dec=Gray  Mapping=[0:15]  PowType=Min. distance between symbols  MinDist=model.parameter.Rectangular_QAM_Demodulator_Baseband.Minimum_distance  AvgPow=1  PeakPow=1  Ph=0  outDtype1=Inherit via internal rule  outDtype2=Inherit via internal rule  derotateFactorWordLen=16  derotateFactorDataTypeStr=Inherit: Same word length as input  derotateFactorLastDataTypeStr=Inherit: Same word length as input  denormFactorWordLen=16  denormFactorDataTypeStr=Inherit: Same word length as input  denormFactorLastDataTypeStr=Inherit: Same word length as input  prodOutWordLen=32  prodOutOverflowMode=Wrap  prodOutRoundingMode=Floor  prodOutOvFlMode=off  prodOutOvFlModeLastStrValue=off  sumWordLen=32
  Out1 : Outport
  wires:
  In1/1 -> Rectangular QAM Demodulator Baseband/1
  Rectangular QAM Demodulator Baseband/1 -> Out1/1  "REData"

== system Simple_Model_Packaging_2/Baseband Signal Selector Rx/If Action Subsystem5 ==
  In1 : Inport
  Action Port : ActionPort  ActionPortLabel=else
  Rectangular QAM Demodulator Baseband : commdigbbndam3/Rectangular QAM Demodulator Baseband  M=model.user_defined.Rectangular_QAM_Modulator_Baseband.M_Number  OutType=Integer  DecType=Hard decision  VarSource=Dialog  Variance=1  Dec=Gray  Mapping=[0:15]  PowType=Min. distance between symbols  MinDist=2  AvgPow=1  PeakPow=1  Ph=0  outDtype1=Inherit via internal rule  outDtype2=Inherit via internal rule  derotateFactorWordLen=16  derotateFactorDataTypeStr=Inherit: Same word length as input  derotateFactorLastDataTypeStr=Inherit: Same word length as input  denormFactorWordLen=16  denormFactorDataTypeStr=Inherit: Same word length as input  denormFactorLastDataTypeStr=Inherit: Same word length as input  prodOutWordLen=32  prodOutOverflowMode=Wrap  prodOutRoundingMode=Floor  prodOutOvFlMode=off  prodOutOvFlModeLastStrValue=off  sumWordLen=32
  Out1 : Outport
  wires:
  In1/1 -> Rectangular QAM Demodulator Baseband/1
  Rectangular QAM Demodulator Baseband/1 -> Out1/1

== system Simple_Model_Packaging_2/Baseband Signal Selector Tx/If Action Subsystem1 ==
  In1 : Inport
  Action Port : ActionPort  ActionPortLabel=elseif(u1 == 2)
  M-PSK Modulator Baseband : commdigbbndpm3/M-PSK Modulator Baseband  M=model.user_defined.Rectangular_QAM_Modulator_Baseband.M_Number  InType=Integer  Enc=Gray  Mapping=[0:7]  Ph=0  outDtype=double  outWordLen=16  outUDDataType=sfix(16)  outFracLenMode=Best precision  outFracLen=15  outDataTypeStr=double  outLastDataTypeStr=double
  Out1 : Outport
  wires:
  M-PSK Modulator Baseband/1 -> Out1/1
  In1/1 -> M-PSK Modulator Baseband/1

== system Simple_Model_Packaging_2/Baseband Signal Selector Tx/If Action Subsystem4 ==
  In1 : Inport
  Action Port : ActionPort  ActionPortLabel=if(u1 == 1)
  Rectangular QAM Modulator Baseband : commdigbbndam3/Rectangular QAM Modulator Baseband  M=model.user_defined.Rectangular_QAM_Modulator_Baseband.M_Number  InType=Integer  Enc=Gray  Mapping=[0:15]  PowType=Min. distance between symbols  MinDist=model.parameter.Rectangular_QAM_Modulator_Baseband.Minimum_distance  AvgPow=1  PeakPow=1  Ph=0  outDtype=double  outWordLen=16  outUDDataType=sfix(16)  outFracLenMode=Best precision  outFracLen=15  outDataTypeStr=double  outLastDataTypeStr=double
      settings: LibrarySourceBlock=|
      | commhdldigbbndam/Rectangular QAM
      | Modulator
      | Baseband
  Out1 : Outport
  wires:
  Rectangular QAM Modulator Baseband/1 -> Out1/1
  In1/1 -> Rectangular QAM Modulator Baseband/1

== system Simple_Model_Packaging_2/Baseband Signal Selector Tx/If Action Subsystem5 ==
  In1 : Inport
  Action Port : ActionPort  ActionPortLabel=else
  Rectangular QAM Modulator Baseband1 : commdigbbndam3/Rectangular QAM Modulator Baseband  M=model.user_defined.Rectangular_QAM_Modulator_Baseband.M_Number  InType=Integer  Enc=Gray  Mapping=[0:15]  PowType=Min. distance between symbols  MinDist=2  AvgPow=1  PeakPow=1  Ph=0  outDtype=double  outWordLen=16  outUDDataType=sfix(16)  outFracLenMode=Best precision  outFracLen=15  outDataTypeStr=double  outLastDataTypeStr=double
      settings: LibrarySourceBlock=|
      | commhdldigbbndam/Rectangular QAM
      | Modulator
      | Baseband
  Out1 : Outport
  wires:
  In1/1 -> Rectangular QAM Modulator Baseband1/1
  Rectangular QAM Modulator Baseband1/1 -> Out1/1

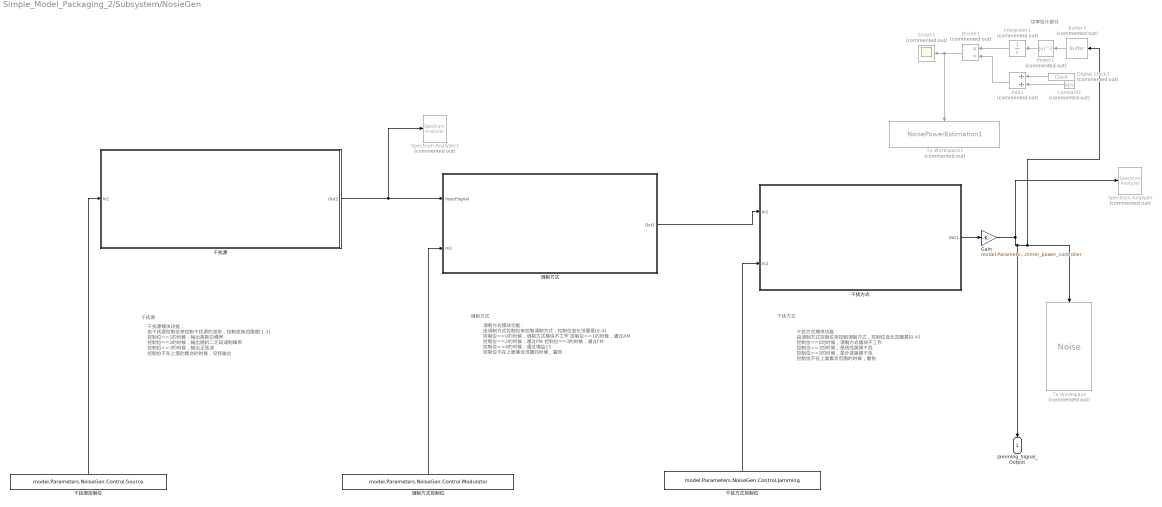
== system Simple_Model_Packaging_2/Subsystem/NosieGen ==
  note: 干扰源
  note: 调制方式
  note: 调制方式模块功能：
      | 由调制方式控制位来控制调制方式，控制位变化范围是[0-4]
      | 控制位==0的时候，调制方式模块不工作
      | 控制位==1的时候，通过AM
      | 控制位==2的时候，通过PM
      | 控制位==3的时候，通过FM
      | 控制位==4的时候，通过增益15
      | 控制位不在上面集合范围的时候，警告
  note: 干扰方式模块功能：
      | 由调制方式控制位来控制调制方式，控制位变化范围是[0-4]
      | 控制位==0的时候，调制方式模块不工作
      | 控制位==1的时候，是线性跳频干扰
      | 控制位==2的时候，是步进跳频干扰
      | 控制位不在上面集合范围的时候，警告
  note: 干扰源模块功能：
      | 由干扰源控制位来控制干扰源的波形，控制变换范围是[1-3]
      | 控制位==1的时候，输出高斯白噪声
      | 控制位==2的时候，输出随机二元码调制噪声
      | 控制位==3的时候，输出正弦波
      | 控制位不在上面的集合的时候，没有输出
  note: 干扰方式
  note: 功率估计部分
  Add1 : Sum  Commented=on
  Buffer7 : Buffer  Commented=on  N=1  OutputFrames=off
  Constant1 : Constant  Commented=on  Value=eps  SampleTime=model.Parameters.NoiseGen.NoiseTs
  Digital Clock1 : DigitalClock  Commented=on  SampleTime=model.Parameters.NoiseGen.NoiseTs
  Divide1 : Product  Commented=on  Inputs=*/
  Gain : Gain  Gain=model.Parameters.jammer_power_controller
  Integrator1 : Integrator  Commented=on
  Power1 : Math  Commented=on  Operator=magnitude^2
  Scope1 : Scope  Commented=on
  Spectrum Analyzer : SpectrumAnalyzer  Commented=on
  Spectrum Analyzer1 : SpectrumAnalyzer  Commented=on
  To Workspace : ToWorkspace  Commented=on  VariableName=Noise  SaveFormat=Timeseries  SampleTime=-1
  To Workspace1 : ToWorkspace  Commented=on  VariableName=NoisePowerEstimation1  SaveFormat=Timeseries  SampleTime=-1
  干扰方式 : Subsystem
  干扰方式控制位 : Constant  Value=model.Parameters.NoiseGen.Control.Jamming  SampleTime=Inf
  干扰源 : Subsystem
  干扰源控制位 : Constant  Value=model.Parameters.NoiseGen.Control.Source  SampleTime=Inf
  调制方式 : Subsystem
  调制方式控制位 : Constant  Value=model.Parameters.NoiseGen.Control.Modulator  SampleTime=Inf
  Jamming_Signal_Output : Outport
  wires:
  Digital Clock1/1 -> Add1/1
  Add1/1 -> Divide1/2
  干扰源控制位/1 -> 干扰源/1(In1)
  Power1/1 -> Integrator1/1
  Gain/1 -> Jamming_Signal_Output/1, Buffer7/1, To Workspace/1, Spectrum Analyzer/1
  Buffer7/1 -> Power1/1
  Divide1/1 -> Scope1/1, To Workspace1/1
  调制方式/1(Out1) -> 干扰方式/1(In1)
  Constant1/1 -> Add1/2
  调制方式控制位/1 -> 调制方式/2(In2)
  干扰源/1(Out1) -> Spectrum Analyzer1/1, 调制方式/1(InputSignal)
  干扰方式控制位/1 -> 干扰方式/2(In2)
  干扰方式/1(Out1) -> Gain/1
  Integrator1/1 -> Divide1/1

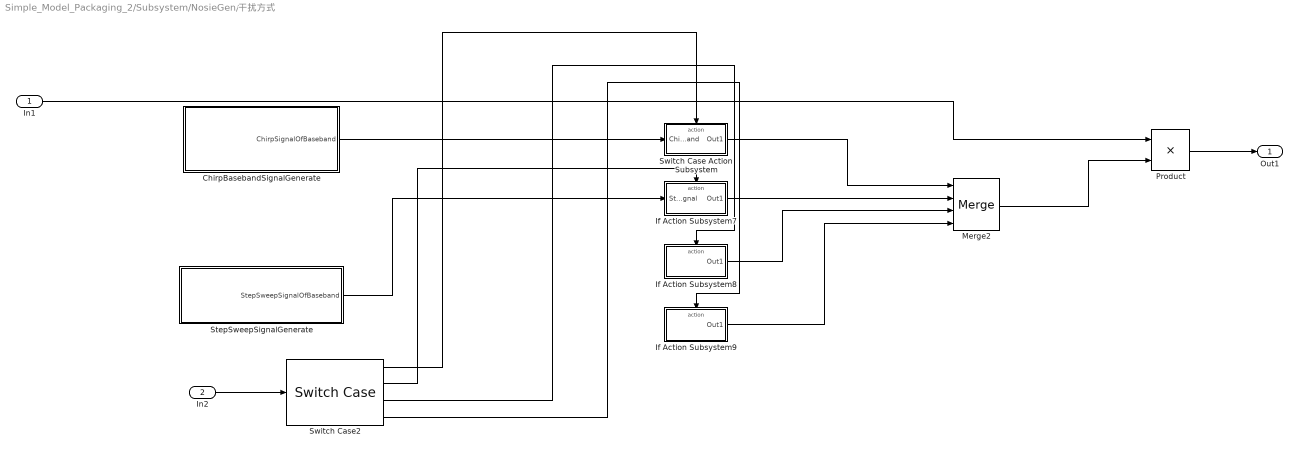
== system Simple_Model_Packaging_2/Subsystem/NosieGen/干扰方式 ==
  In1 : Inport
  In2 : Inport  Port=2
  ChirpBasebandSignalGenerate : Subsystem
      settings: AttributesFormatString=|
      | 线性调频模块：线性调频公式(y=exp(2*pi*(f_min*t+0.5*k_chirp*t^2)))
      | 输入参数：
      | 1. f_min,为线性调频信号的起始频率
      | 2.f_max为线性调频信号的终止频率
      | 3.T_chirp为线性调频信号的调频时间
      | 斜率k_sweep = (f_min-f_max)/T_chirp
  If Action Subsystem7 : Subsystem  TreatAsAtomicUnit=on
  If Action Subsystem8 : Subsystem  TreatAsAtomicUnit=on
  If Action Subsystem9 : Subsystem  TreatAsAtomicUnit=on
  Merge2 : Merge  Inputs=4
  Product : Product
  StepSweepSignalGenerate : Subsystem
  Switch Case Action Subsystem : Subsystem  TreatAsAtomicUnit=on
  Switch Case2 : SwitchCase  CaseConditions={1,2,3}
  Out1 : Outport
  wires:
  If Action Subsystem9/1(Out1) -> Merge2/4
  Switch Case Action Subsystem/1(Out1) -> Merge2/1
  If Action Subsystem8/1(Out1) -> Merge2/3
  Switch Case2/3 -> If Action Subsystem8/Action
  Switch Case2/1 -> Switch Case Action Subsystem/Action
  Switch Case2/2 -> If Action Subsystem7/Action
  Switch Case2/4 -> If Action Subsystem9/Action
  ChirpBasebandSignalGenerate/1(ChirpSignalOfBaseband) -> Switch Case Action Subsystem/1(ChirpSignalOfBaseband)
  If Action Subsystem7/1(Out1) -> Merge2/2
  Merge2/1 -> Product/2
  Product/1 -> Out1/1
  In1/1 -> Product/1
  In2/1 -> Switch Case2/1
  StepSweepSignalGenerate/1(StepSweepSignalOfBaseband) -> If Action Subsystem7/1(StepSweepSignal)

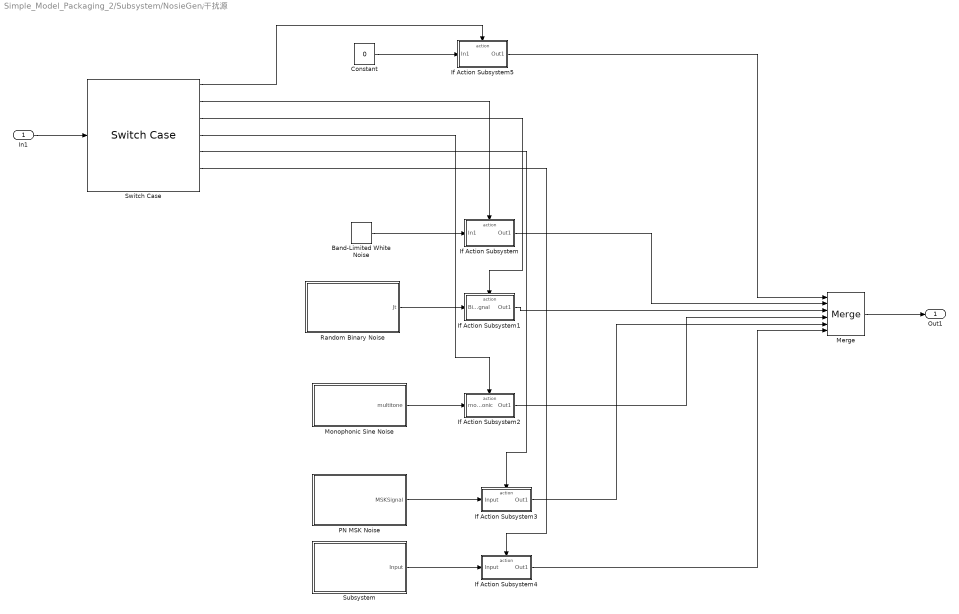
== system Simple_Model_Packaging_2/Subsystem/NosieGen/干扰源 ==
  In1 : Inport
  Band-Limited White Noise : simulink/Sources/Band-Limited White Noise  Cov=model.Parameters.NoiseGen.GaussPower  Ts=model.Parameters.NoiseGen.NoiseTs  seed=model.Parameters.NoiseGen.GaussSeed
  Constant : Constant  Value=0  SampleTime=model.Parameters.NoiseGen.NoiseTs
  If Action Subsystem : Subsystem  TreatAsAtomicUnit=on
  If Action Subsystem1 : Subsystem  TreatAsAtomicUnit=on
  If Action Subsystem2 : Subsystem  TreatAsAtomicUnit=on
  If Action Subsystem3 : Subsystem  TreatAsAtomicUnit=on
  If Action Subsystem4 : Subsystem  TreatAsAtomicUnit=on
  If Action Subsystem5 : Subsystem  TreatAsAtomicUnit=on
  Merge : Merge  Inputs=6
  Monophonic Sine Noise : Subsystem
  PN MSK Noise : Subsystem
  Random Binary Noise : Subsystem
  Subsystem : Subsystem
  Switch Case : SwitchCase  CaseConditions={0,1,2,3,4,5}
  Out1 : Outport
  wires:
  Switch Case/3 -> If Action Subsystem1/Action
  If Action Subsystem2/1(Out1) -> Merge/4
  Band-Limited White Noise/1 -> If Action Subsystem/1(In1)
  If Action Subsystem1/1(Out1) -> Merge/3
  Random Binary Noise/1(Jt) -> If Action Subsystem1/1(Binary_Random_Signal)
  Switch Case/4 -> If Action Subsystem2/Action
  Switch Case/2 -> If Action Subsystem/Action
  Merge/1 -> Out1/1
  In1/1 -> Switch Case/1
  Monophonic Sine Noise/1(multitone) -> If Action Subsystem2/1(monophonic)
  Switch Case/5 -> If Action Subsystem3/Action
  If Action Subsystem3/1(Out1) -> Merge/5
  If Action Subsystem/1(Out1) -> Merge/2
  PN MSK Noise/1(MSKSignal) -> If Action Subsystem3/1(Input)
  Switch Case/6 -> If Action Subsystem4/Action
  Subsystem/1(Input) -> If Action Subsystem4/1(Input)
  If Action Subsystem4/1(Out1) -> Merge/6
  Switch Case/1 -> If Action Subsystem5/Action
  Constant/1 -> If Action Subsystem5/1(In1)
  If Action Subsystem5/1(Out1) -> Merge/1

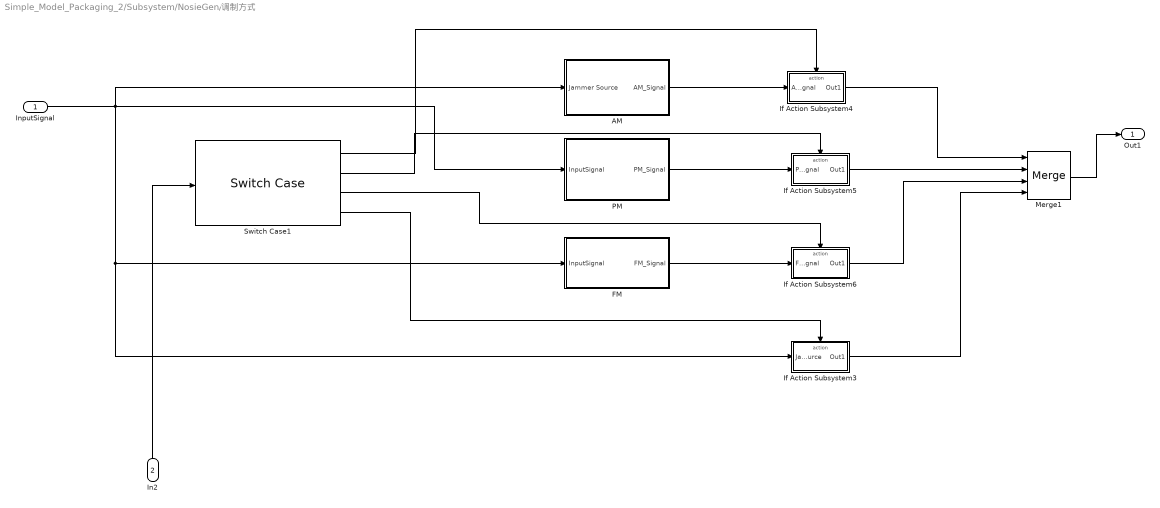
== system Simple_Model_Packaging_2/Subsystem/NosieGen/调制方式 ==
  InputSignal : Inport
  In2 : Inport  Port=2
  AM : Subsystem
  FM : Subsystem
  If Action Subsystem3 : Subsystem  TreatAsAtomicUnit=on
  If Action Subsystem4 : Subsystem  TreatAsAtomicUnit=on
  If Action Subsystem5 : Subsystem  TreatAsAtomicUnit=on
  If Action Subsystem6 : Subsystem  TreatAsAtomicUnit=on
  Merge1 : Merge  Inputs=4
  PM : Subsystem
  Switch Case1 : SwitchCase  CaseConditions={1,2,3}
  Out1 : Outport
  wires:
  In2/1 -> Switch Case1/1
  PM/1(PM_Signal) -> If Action Subsystem5/1(PM_Signal)
  Merge1/1 -> Out1/1
  If Action Subsystem3/1(Out1) -> Merge1/4
  If Action Subsystem6/1(Out1) -> Merge1/3
  If Action Subsystem5/1(Out1) -> Merge1/2
  InputSignal/1 -> FM/1(InputSignal), If Action Subsystem3/1(Jammer Source), PM/1(InputSignal), AM/1(Jammer Source)
  AM/1(AM_Signal) -> If Action Subsystem4/1(AM_Signal)
  Switch Case1/2 -> If Action Subsystem5/Action
  Switch Case1/3 -> If Action Subsystem6/Action
  Switch Case1/1 -> If Action Subsystem4/Action
  If Action Subsystem4/1(Out1) -> Merge1/1
  FM/1(FM_Signal) -> If Action Subsystem6/1(FM_Signal)
  Switch Case1/4 -> If Action Subsystem3/Action

== system Simple_Model_Packaging_2/Subsystem/NosieGen/干扰方式/ChirpBasebandSignalGenerate ==
  note: 线性调频模块：线性调频公式(y=exp(2*pi*(fmin*t+0.5*k_chirp*t^2)))
      | 输入参数：
      | 1.fmin,为线性调频信号的起始频率
      | 2.fmax为线性调频信号的终止频率
      | 3.T_chirp为线性调频信号的调频时间
      | 斜率k_sweep = (f_min-f_max)/T_chirp
  note: 线性调频模块
  Chirp_Signal_Generation : MATLAB Function  TreatAsAtomicUnit=on
  Constant : Constant  Value=model.Parameters.NoiseGen.Jamming.LinearSweepFmin
  Constant1 : Constant  Value=model.Parameters.NoiseGen.Jamming.LinearSweepT
  Constant2 : Constant  Value=model.Parameters.NoiseGen.Jamming.LinearSweepK
  Digital Clock : DigitalClock  SampleTime=model.Parameters.NoiseGen.NoiseTs
  Frequency_Check : Subsystem  Commented=on
  ChirpSignalOfBaseband : Outport
  wires:
  Digital Clock/1 -> Chirp_Signal_Generation/1(t)
  Chirp_Signal_Generation/1(y) -> ChirpSignalOfBaseband/1  "ChirpSignal"
  Frequency_Check/1(FrequencyConversionLine) -> ?
  Constant/1 -> Chirp_Signal_Generation/2(f_chirp_min)
  Constant2/1 -> Chirp_Signal_Generation/4(k_chirp)
  Constant1/1 -> Chirp_Signal_Generation/3(T_chirp)

== system Simple_Model_Packaging_2/Subsystem/NosieGen/干扰方式/If Action Subsystem7 ==
  StepSweepSignal : Inport
  Action Port : ActionPort  ActionPortLabel=case [ 2 ]:
  Out1 : Outport
  wires:
  StepSweepSignal/1 -> Out1/1

== system Simple_Model_Packaging_2/Subsystem/NosieGen/干扰方式/If Action Subsystem8 ==
  Action Port : ActionPort  ActionPortLabel=case [ 3 ]:
  Constant : Constant  Value=10
  Constant1 : Constant  Value=0
  Real-Imag to Complex : RealImagToComplex
  Out1 : Outport
  wires:
  Constant/1 -> Real-Imag to Complex/1
  Real-Imag to Complex/1 -> Out1/1
  Constant1/1 -> Real-Imag to Complex/2

== system Simple_Model_Packaging_2/Subsystem/NosieGen/干扰方式/If Action Subsystem9 ==
  Action Port : ActionPort  ActionPortLabel=default:
  Constant : Constant
  Constant1 : Constant  Value=0
  Real-Imag to Complex : RealImagToComplex
  Out1 : Outport
  wires:
  Constant/1 -> Real-Imag to Complex/1
  Real-Imag to Complex/1 -> Out1/1
  Constant1/1 -> Real-Imag to Complex/2

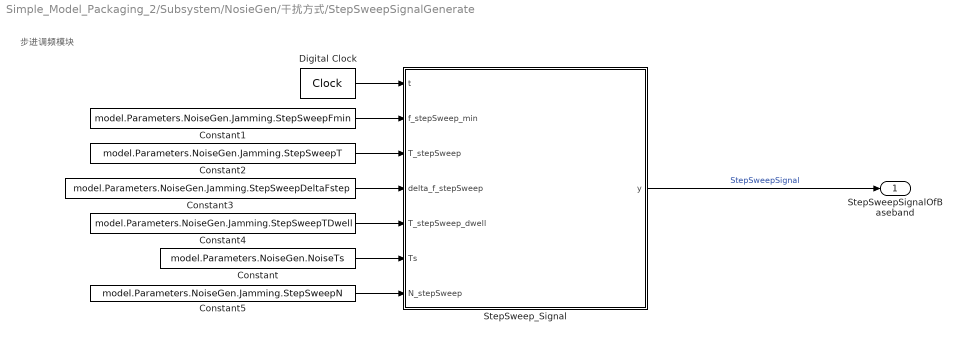
== system Simple_Model_Packaging_2/Subsystem/NosieGen/干扰方式/StepSweepSignalGenerate ==
  note: 步进调频模块
  Constant : Constant  Value=model.Parameters.NoiseGen.NoiseTs
  Constant1 : Constant  Value=model.Parameters.NoiseGen.Jamming.StepSweepFmin
  Constant2 : Constant  Value=model.Parameters.NoiseGen.Jamming.StepSweepT
  Constant3 : Constant  Value=model.Parameters.NoiseGen.Jamming.StepSweepDeltaFstep
  Constant4 : Constant  Value=model.Parameters.NoiseGen.Jamming.StepSweepTDwell
  Constant5 : Constant  Value=model.Parameters.NoiseGen.Jamming.StepSweepN
  Digital Clock : DigitalClock  SampleTime=model.Parameters.NoiseGen.NoiseTs
  StepSweep_Signal : MATLAB Function  TreatAsAtomicUnit=on
  StepSweepSignalOfBaseband : Outport
  wires:
  Digital Clock/1 -> StepSweep_Signal/1(t)
  StepSweep_Signal/1(y) -> StepSweepSignalOfBaseband/1  "StepSweepSignal"
  Constant/1 -> StepSweep_Signal/6(Ts)
  Constant1/1 -> StepSweep_Signal/2(f_stepSweep_min)
  Constant2/1 -> StepSweep_Signal/3(T_stepSweep)
  Constant3/1 -> StepSweep_Signal/4(delta_f_stepSweep)
  Constant4/1 -> StepSweep_Signal/5(T_stepSweep_dwell)
  Constant5/1 -> StepSweep_Signal/7(N_stepSweep)

== system Simple_Model_Packaging_2/Subsystem/NosieGen/干扰方式/Switch Case Action Subsystem ==
  ChirpSignalOfBaseband : Inport
  Action Port : ActionPort  ActionPortLabel=case [ 1 ]:
  Out1 : Outport
  wires:
  ChirpSignalOfBaseband/1 -> Out1/1
